simulink model "Heli_LQR2"  (Simulink 6.3)
settings: Solver=ode1  SolverMode=SingleTasking  StartTime=0.0  StopTime=inf  FixedStep=0.001  RelTol=1e-3
values from neighbouring files (symbols this model uses):
  g = 9.81    [setup_heli_LQR_instructor.m]    (also in setup_heli_LQR_parameters.m)
  h = 0.0139    [setup_heli_LQR_instructor.m]    (also in setup_heli_LQR_parameters.m)
  INT_JOYSTICK_SAT_LOWER = theta_0 * 180 / pi    (= -30)    [setup_heli_LQR_instructor.m]    (also in setup_heli_LQR_parameters.m)
  INT_JOYSTICK_SAT_UPPER = abs(theta_0)  * 180 / pi    [setup_heli_LQR_instructor.m]    (also in setup_heli_LQR_parameters.m)
  JOYSTICK_X_DZ = 0.25    [setup_heli_LQR_instructor.m]    (also in setup_heli_LQR_parameters.m)
  JOYSTICK_Y_DZ = 0.25    [setup_heli_LQR_instructor.m]    (also in setup_heli_LQR_parameters.m)
  K_CABLE_P = 5    [setup_heli_LQR_instructor.m]    (also in setup_heli_LQR_parameters.m)
  K_CABLE_Y = 3    [setup_heli_LQR_instructor.m]    (also in setup_heli_LQR_parameters.m)
  K_EC_P = - 2 * pi / ( 4 * 1024 )    (= -0.00153398078789)    [setup_heli_LQR_instructor.m]    (also in setup_heli_LQR_parameters.m)
  K_EC_Y = 2 * pi / ( 8 * 1024 )    (= 0.000766990393943)    [setup_heli_LQR_instructor.m]    (also in setup_heli_LQR_parameters.m)
  K_JOYSTICK_X = 85    [setup_heli_LQR_instructor.m]    (also in setup_heli_LQR_parameters.m)
  K_JOYSTICK_Y = 85    [setup_heli_LQR_instructor.m]    (also in setup_heli_LQR_parameters.m)
  K_pp = 0.185*0.20962    (= 0.0387797)    [setup_heli_LQR_instructor.m]    (also in setup_heli_LQR_parameters.m)
  K_py = 0.0041362    [setup_heli_LQR_instructor.m]    (also in setup_heli_LQR_parameters.m)
  K_yp = 0.0083316    [setup_heli_LQR_instructor.m]    (also in setup_heli_LQR_parameters.m)
  K_yy = 0.185*0.050271    (= 0.009300135)    [setup_heli_LQR_instructor.m]    (also in setup_heli_LQR_parameters.m)
  Ki = lqr(a,b,Qi,R)    [setup_heli_LQR_instructor.m]
  m_heli = 1.326    [setup_heli_LQR_instructor.m]    (also in setup_heli_LQR_parameters.m)
  Rc = 0.0094    [setup_heli_LQR_instructor.m]    (also in setup_heli_LQR_parameters.m)
  SAT_INT_ERR_PITCH = 20    [setup_heli_LQR_instructor.m]    (also in setup_heli_LQR_parameters.m)
  SAT_INT_ERR_YAW = 20    [setup_heli_LQR_instructor.m]    (also in setup_heli_LQR_parameters.m)
  theta_0 = -30*pi/180    (= -0.523598775598)    [setup_heli_LQR_instructor.m]    (also in setup_heli_LQR_parameters.m)
  Tr_p = 1    [setup_heli_LQR_instructor.m]    (also in setup_heli_LQR_parameters.m)
  Tr_y = 1    [setup_heli_LQR_instructor.m]    (also in setup_heli_LQR_parameters.m)
  VMAX_DAC = 10    [setup_heli_LQR_instructor.m]    (also in setup_heli_LQR_parameters.m)
  VMAX_UPM_P = 24    [setup_heli_LQR_instructor.m]    (also in setup_heli_LQR_parameters.m)
  VMAX_UPM_Y = 15    [setup_heli_LQR_instructor.m]    (also in setup_heli_LQR_parameters.m)
  wcf = 2 * pi * 20    (= 125.663706144)    [setup_heli_LQR_instructor.m]    (also in setup_heli_LQR_parameters.m)
  zetaf = 0.85    [setup_heli_LQR_instructor.m]    (also in setup_heli_LQR_parameters.m)
undefined symbols (not defined in the file or in its folder): Joystick, q_modules3
libraries: qctools x3
settings Model: LastModifiedBy=localadmin  ExtModeArmWhenConnect=off  BufferReuse=off  StrictBusMsg=None
settings ConfigSet: SimulationMode=external
settings OptimizationCC: BooleanDataType=off  InlineInvariantSignals=on  OptimizeBlockIOStorage=off  BufferReuse=off  ExpressionFolding=off  LocalBlockOutputs=off
settings RTWCC: SystemTargetFile=wincon.tlc  MakeCommand=make_wc  TemplateMakefile=wc_default_tmf  Description=WinCon Target  ProcessScript=wincon_make_rtw_hook
settings STFCustomTargetCC: TargetFcnLib=ansi_tfl_tmw.mat  GenFloatMathFcnCalls=ANSI_C  ModelReferenceCompliant=off  SystemTargetFile=wincon.tlc
settings GRTTargetCC: ModelReferenceCompliant=off  MatFileLogging=off  ExtMode=on  ExtModeTransport=2  ExtModeMexFile=wc_comm
settings CustomProperty: Value=on

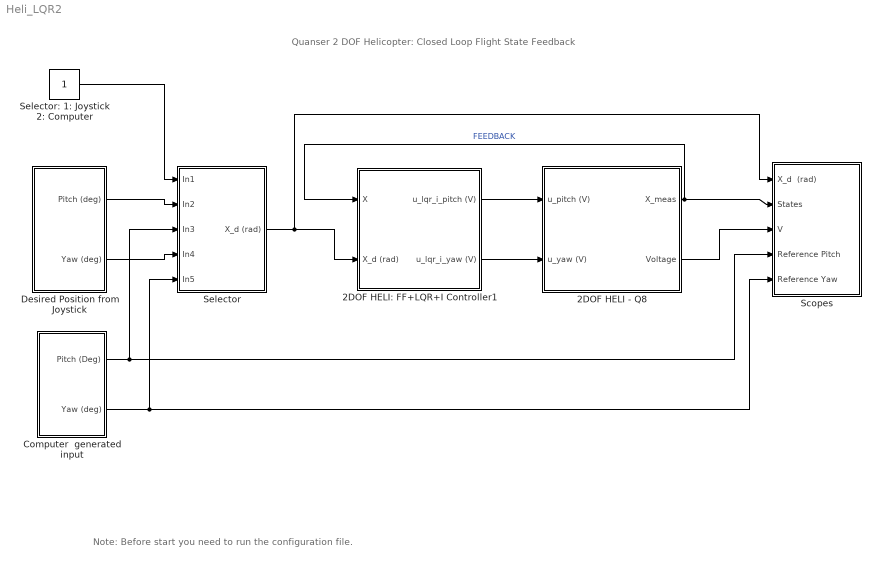
== system Heli_LQR2 ==
  note: Quanser 2 DOF Helicopter:
      | Closed Loop Flight
      | State Feedback
  note: Note: Before start you need to run the configuration file.
  2DOF HELI - Q8 : Subsystem  AncestorBlock=heli_2d_lib/2DOF HELI - Q8
  2DOF HELI: FF+LQR+I Controller1 : Subsystem  AncestorBlock=heli_2d_lib/2DOF HELI: FF+LQR+I Controller
  Computer  generated input : Subsystem
  Desired Position from Joystick : Subsystem  AncestorBlock=q_modules3/Joystick
  Scopes : Subsystem
  Selector : Subsystem
  Selector: 1: Joystick 2: Computer : Constant
  wires:
  2DOF HELI - Q8/1(X_meas) -> Scopes/2(States), 2DOF HELI: FF+LQR+I Controller1/1(X)  "FEEDBACK"
  2DOF HELI: FF+LQR+I Controller1/1(u_lqr_i_pitch (V)) -> 2DOF HELI - Q8/1(u_pitch (V))
  2DOF HELI: FF+LQR+I Controller1/2(u_lqr_i_yaw (V)) -> 2DOF HELI - Q8/2(u_yaw (V))
  Desired Position from Joystick/1(Pitch (deg)) -> Selector/2(In2)
  Computer  generated input/1(Pitch (Deg)) -> Selector/3(In3), Scopes/4(Reference Pitch)
  Desired Position from Joystick/2(Yaw (deg)) -> Selector/4(In4)
  Computer  generated input/2(Yaw (deg)) -> Selector/5(In5), Scopes/5(Reference Yaw)
  Selector: 1: Joystick 2: Computer/1 -> Selector/1(In1)
  Selector/1(X_d (rad)) -> Scopes/1(X_d  (rad)), 2DOF HELI: FF+LQR+I Controller1/2(X_d (rad))
  2DOF HELI - Q8/2(Voltage) -> Scopes/3(V)

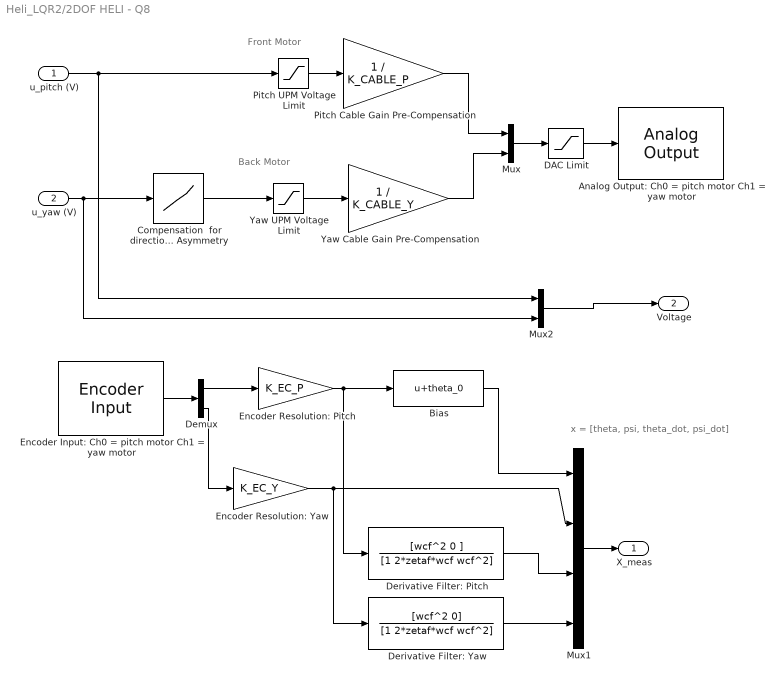
== system Heli_LQR2/2DOF HELI - Q8 ==
  note: Back Motor
  note: Front Motor
  note: x = [theta, psi, theta_dot, psi_dot]
  u_pitch (V) : Inport
  u_yaw (V) : Inport  Port=2
  Analog Output: Ch0 = pitch motor Ch1 = yaw motor : qctools/Quanser Consulting Q8 Series/Analog Output  boardNumber=0  channels=[0,1]  modesVect=0  rangesVect=10  initialVect=0  finalVect=0  sampleTime=-1  inputVolts=on  simulationOutput=off
  Bias : Bias  Bias=theta_0
  "Compensation  for direction Asymmetry " : Lookup  InputValues="[-[12.5  10 7.5]  0  [7.5 10  12.5 15] ]"  OutputValues="[-[12.5  10 7.5] *.4 0  [7.5 10  12.5 15] ]"
  DAC Limit : Saturate  UpperLimit=VMAX_DAC  LowerLimit=- VMAX_DAC
  Demux : Demux  Outputs=2
  Derivative Filter: Pitch : TransferFcn  Numerator=[wcf^2 0 ]  Denominator=[1 2*zetaf*wcf wcf^2]
  Derivative Filter: Yaw : TransferFcn  Numerator=[wcf^2 0]  Denominator=[1 2*zetaf*wcf wcf^2]
  Encoder Input: Ch0 = pitch motor Ch1 = yaw motor : qctools/Quanser Consulting Q8 Series/Encoder Input  boardNumber=0  channels=[0,1]  initial=0  preserveCounts=off  sampleTime=default_sample_time  quadratureStr=4X  modeStr=Normal  flagString=FLG1 is IDX and FLG2 is E  prescale=1  frequency=16666666.6667  bcd=off  enableIndex=on  synchronousIndex=on  indexPolarity=on  reloadOnIndex=off  simulationInput=off
  "Encoder Resolution: Pitch " : Gain  Gain=K_EC_P
  Encoder Resolution: Yaw : Gain  Gain=K_EC_Y
  Mux : Mux  Inputs=2
  Mux1 : Mux
  Mux2 : Mux  Inputs=2
  Pitch Cable Gain Pre-Compensation : Gain  Gain=1 / K_CABLE_P  SaturateOnIntegerOverflow=on
  Pitch UPM Voltage Limit : Saturate  UpperLimit=VMAX_UPM_P  LowerLimit=- VMAX_UPM_P
  Yaw Cable Gain Pre-Compensation : Gain  Gain=1 / K_CABLE_Y  SaturateOnIntegerOverflow=on
  Yaw UPM Voltage Limit : Saturate  UpperLimit=VMAX_UPM_Y  LowerLimit=- VMAX_UPM_Y
  X_meas : Outport
  Voltage : Outport  Port=2
  wires:
  Encoder Resolution: Yaw/1 -> Mux1/2, Derivative Filter: Yaw/1
  Yaw Cable Gain Pre-Compensation/1 -> Mux/2
  Pitch Cable Gain Pre-Compensation/1 -> Mux/1
  Mux1/1 -> X_meas/1
  u_pitch (V)/1 -> Pitch UPM Voltage Limit/1, Mux2/1
  Yaw UPM Voltage Limit/1 -> Yaw Cable Gain Pre-Compensation/1
  Pitch UPM Voltage Limit/1 -> Pitch Cable Gain Pre-Compensation/1
  DAC Limit/1 -> Analog Output: Ch0 = pitch motor Ch1 = yaw motor/1
  Mux/1 -> DAC Limit/1
  Demux/1 -> "Encoder Resolution: Pitch "/1
  "Encoder Resolution: Pitch "/1 -> Bias/1, Derivative Filter: Pitch/1
  Encoder Input: Ch0 = pitch motor Ch1 = yaw motor/1 -> Demux/1
  Demux/2 -> Encoder Resolution: Yaw/1
  Bias/1 -> Mux1/1
  Derivative Filter: Pitch/1 -> Mux1/3
  Derivative Filter: Yaw/1 -> Mux1/4
  "Compensation  for direction Asymmetry "/1 -> Yaw UPM Voltage Limit/1
  u_yaw (V)/1 -> "Compensation  for direction Asymmetry "/1, Mux2/2
  Mux2/1 -> Voltage/1

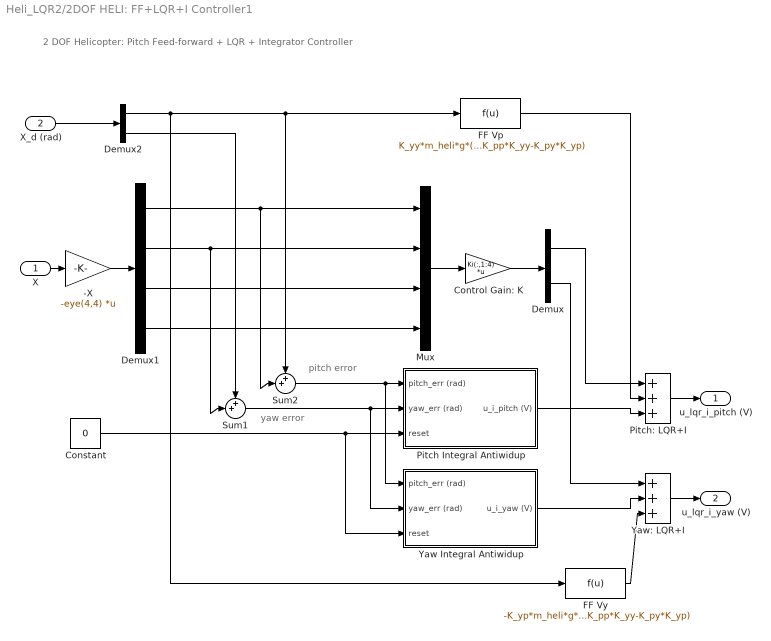
== system Heli_LQR2/2DOF HELI: FF+LQR+I Controller1 ==
  note: yaw error
  note: pitch error
  note: 2 DOF Helicopter:
      | Pitch Feed-forward + LQR + Integrator Controller
  X : Inport
  X_d (rad) : Inport  Port=2
  -X : Gain  Gain=-eye(4,4)  Multiplication=Matrix(K*u)
  Constant : Constant  Value=0
  Control Gain: K : Gain  Gain=Ki(:,1:4)  Multiplication=Matrix(K*u)
  Demux : Demux  Outputs=2
  Demux1 : Demux
  Demux2 : Demux  Outputs=2
  FF Vp : Fcn  Expr="K_yy*m_heli*g*(h*sin(u[1]) + Rc*cos(u[1]))  /  (K_pp*K_yy-K_py*K_yp)"
  FF Vy : Fcn  Expr="-K_yp*m_heli*g*(h*sin(u[1]) + Rc*cos(u[1]))  /  (K_pp*K_yy-K_py*K_yp)"
  Mux : Mux
  Pitch Integral Antiwidup : Subsystem  AncestorBlock=heli_2d_lib/2DOF HELI: FF+LQR+I Controller/Yaw Integral Antiwidup
  Pitch: LQR+I : Sum  Inputs=+++  OutScaling=2^-10
  Sum1 : Sum  Inputs=++|
  Sum2 : Sum  Inputs=++|
  Yaw Integral Antiwidup : Subsystem
  Yaw: LQR+I : Sum  Inputs=+++  OutScaling=2^-10
  u_lqr_i_pitch (V) : Outport
  u_lqr_i_yaw (V) : Outport  Port=2
  wires:
  Constant/1 -> Pitch Integral Antiwidup/3(reset), Yaw Integral Antiwidup/3(reset)
  Demux1/2 -> Sum1/2, Mux/2
  Demux2/2 -> Sum1/1
  Demux2/1 -> Sum2/1, FF Vp/1, FF Vy/1
  X_d (rad)/1 -> Demux2/1
  Yaw Integral Antiwidup/1(u_i_yaw (V)) -> Yaw: LQR+I/2
  Demux/2 -> Yaw: LQR+I/1
  Yaw: LQR+I/1 -> u_lqr_i_yaw (V)/1
  Pitch: LQR+I/1 -> u_lqr_i_pitch (V)/1
  Demux/1 -> Pitch: LQR+I/2
  Pitch Integral Antiwidup/1(u_i_pitch (V)) -> Pitch: LQR+I/3
  FF Vp/1 -> Pitch: LQR+I/1
  Sum2/1 -> Pitch Integral Antiwidup/1(pitch_err (rad)), Yaw Integral Antiwidup/1(pitch_err (rad))
  Demux1/1 -> Sum2/2, Mux/1
  X/1 -> -X/1
  Sum1/1 -> Pitch Integral Antiwidup/2(yaw_err (rad)), Yaw Integral Antiwidup/2(yaw_err (rad))
  -X/1 -> Demux1/1
  Control Gain: K/1 -> Demux/1
  Mux/1 -> Control Gain: K/1
  Demux1/3 -> Mux/3
  Demux1/4 -> Mux/4
  FF Vy/1 -> Yaw: LQR+I/3

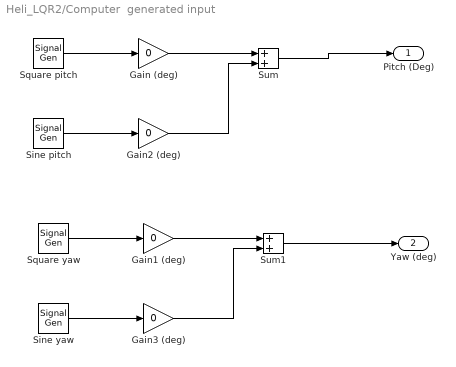
== system Heli_LQR2/Computer  generated input ==
  Gain (deg) : Gain  Gain=0
  Gain1 (deg) : Gain  Gain=0
  Gain2 (deg) : Gain  Gain=0
  Gain3 (deg) : Gain  Gain=0
  Sine pitch : SignalGenerator  Frequency=1/30
  Sine yaw : SignalGenerator  Frequency=.02
  Square pitch : SignalGenerator  WaveForm=square  Frequency=1/30
  Square yaw : SignalGenerator  WaveForm=square  Frequency=1/60*2
  Sum : Sum
  Sum1 : Sum
  Pitch (Deg) : Outport
  Yaw (deg) : Outport  Port=2
  wires:
  Square pitch/1 -> Gain (deg)/1
  Gain (deg)/1 -> Sum/1
  Sum/1 -> Pitch (Deg)/1
  Sine pitch/1 -> Gain2 (deg)/1
  Gain2 (deg)/1 -> Sum/2
  Square yaw/1 -> Gain1 (deg)/1
  Gain1 (deg)/1 -> Sum1/1
  Sum1/1 -> Yaw (deg)/1
  Sine yaw/1 -> Gain3 (deg)/1
  Gain3 (deg)/1 -> Sum1/2

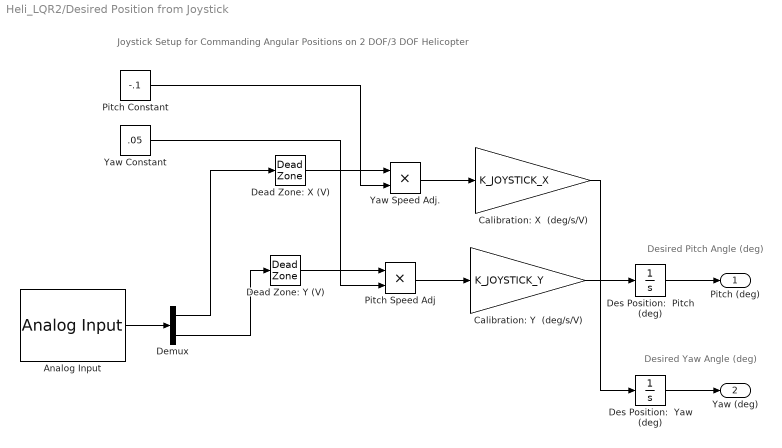
== system Heli_LQR2/Desired Position from Joystick ==
  note: Joystick Setup for Commanding Angular Positions on 2 DOF/3 DOF Helicopter
  note: Desired Yaw Angle (deg)
  note: Desired Pitch Angle (deg)
  Analog Input : qctools/Quanser Consulting Q8 Series/Analog Input  boardNumber=0  channels=[2 3]  sampleTime=default_sample_time  useBusy=on  simultaneous=on  outputVolts=on  simulationInput=off
  Calibration: X  (deg/s/V) : Gain  Gain=K_JOYSTICK_X
  Calibration: Y  (deg/s/V) : Gain  Gain=K_JOYSTICK_Y
  Dead Zone: X (V) : DeadZone  LowerValue=-JOYSTICK_X_DZ  UpperValue=JOYSTICK_X_DZ  SaturateOnIntegerOverflow=on
  Dead Zone: Y (V) : DeadZone  LowerValue=-JOYSTICK_Y_DZ  UpperValue=JOYSTICK_Y_DZ  SaturateOnIntegerOverflow=on
  Demux : Demux  Outputs=2
  Des Position:  Pitch (deg) : Integrator  InitialCondition=theta_0*180/pi  LimitOutput=on  UpperSaturationLimit=INT_JOYSTICK_SAT_UPPER  LowerSaturationLimit=INT_JOYSTICK_SAT_LOWER
  Des Position:  Yaw (deg) : Integrator  UpperSaturationLimit=180  LowerSaturationLimit=-180
  Pitch Constant : Constant  Value=-.1
  Pitch Speed Adj : Product  RndMeth=Zero
  Yaw Constant : Constant  Value=.05
  Yaw Speed Adj. : Product  RndMeth=Zero
  Pitch (deg) : Outport
  Yaw (deg) : Outport  Port=2
  wires:
  Yaw Constant/1 -> Pitch Speed Adj/2
  Demux/2 -> Dead Zone: Y (V)/1
  Demux/1 -> Dead Zone: X (V)/1
  Pitch Constant/1 -> Yaw Speed Adj./2
  Analog Input/1 -> Demux/1
  Calibration: Y  (deg/s/V)/1 -> Des Position:  Pitch (deg)/1
  Pitch Speed Adj/1 -> Calibration: Y  (deg/s/V)/1
  Yaw Speed Adj./1 -> Calibration: X  (deg/s/V)/1
  Dead Zone: Y (V)/1 -> Pitch Speed Adj/1
  Dead Zone: X (V)/1 -> Yaw Speed Adj./1
  Calibration: X  (deg/s/V)/1 -> Des Position:  Yaw (deg)/1
  Des Position:  Yaw (deg)/1 -> Yaw (deg)/1
  Des Position:  Pitch (deg)/1 -> Pitch (deg)/1

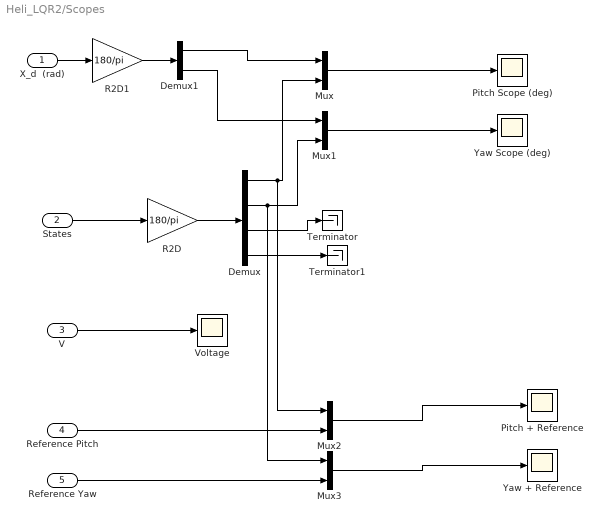
== system Heli_LQR2/Scopes ==
  X_d  (rad) : Inport
  States : Inport  Port=2
  V : Inport  Port=3
  Reference Pitch : Inport  Port=4
  Reference Yaw : Inport  Port=5
  Demux : Demux
  Demux1 : Demux  Outputs=2
  Mux{,1..3} (4 alike) : Mux  Inputs=2
  Pitch + Reference : Scope
  Pitch Scope (deg) : Scope
      settings: SaveName=ScopeData6
  R2D : Gain  Gain=180/pi
  R2D1 : Gain  Gain=180/pi
  Terminator : Terminator
  Terminator1 : Terminator
  Voltage : Scope
  Yaw + Reference : Scope
      settings: SaveName=ScopeData2
  Yaw Scope (deg) : Scope
      settings: SaveName=ScopeData7
  wires:
  Demux/1 -> Mux/2, Mux2/1
  States/1 -> R2D/1
  R2D/1 -> Demux/1
  Mux/1 -> Pitch Scope (deg)/1
  Mux1/1 -> Yaw Scope (deg)/1
  Demux/2 -> Mux1/2, Mux3/1
  Demux/3 -> Terminator/1
  Demux/4 -> Terminator1/1
  X_d  (rad)/1 -> R2D1/1
  Demux1/1 -> Mux/1
  Demux1/2 -> Mux1/1
  R2D1/1 -> Demux1/1
  V/1 -> Voltage/1
  Reference Pitch/1 -> Mux2/2
  Reference Yaw/1 -> Mux3/2
  Mux2/1 -> Pitch + Reference/1
  Mux3/1 -> Yaw + Reference/1

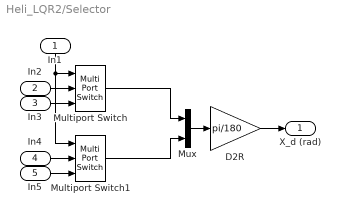
== system Heli_LQR2/Selector ==
  In1 : Inport  Orientation=down
  In2 : Inport  Port=2
  In3 : Inport  Port=3
  In4 : Inport  Port=4
  In5 : Inport  Port=5
  D2R : Gain  Gain=pi/180
  Multiport Switch : MultiPortSwitch  Inputs=2
  Multiport Switch1 : MultiPortSwitch  Inputs=2
  Mux : Mux  Inputs=2
  X_d (rad) : Outport
  wires:
  In1/1 -> Multiport Switch/1, Multiport Switch1/1
  In2/1 -> Multiport Switch/2
  Multiport Switch/1 -> Mux/1
  In3/1 -> Multiport Switch/3
  In4/1 -> Multiport Switch1/2
  Multiport Switch1/1 -> Mux/2
  In5/1 -> Multiport Switch1/3
  Mux/1 -> D2R/1
  D2R/1 -> X_d (rad)/1

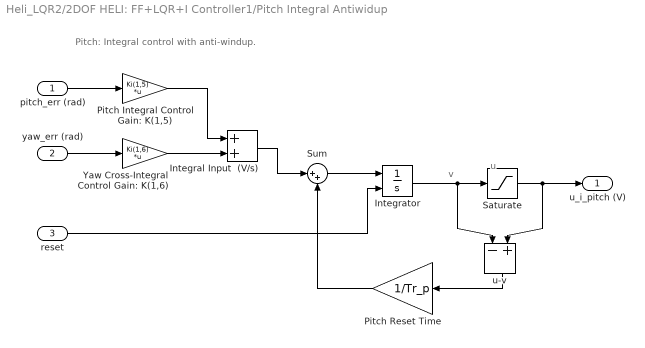
== system Heli_LQR2/2DOF HELI: FF+LQR+I Controller1/Pitch Integral Antiwidup ==
  note: Pitch: Integral control with anti-windup.
  note: v
  note: u
  pitch_err (rad) : Inport
  yaw_err (rad) : Inport  Port=2
  reset : Inport  Port=3
  Integral Input  (V/s) : Sum  OutScaling=2^-10
  Integrator : Integrator  ExternalReset=rising
  Pitch Integral Control Gain: K(1,5) : Gain  Gain=Ki(1,5)  Multiplication=Matrix(K*u)
  Pitch Reset Time : Gain  Orientation=left  Gain=1/Tr_p
  Saturate : Saturate  UpperLimit=SAT_INT_ERR_PITCH  LowerLimit=-SAT_INT_ERR_PITCH
  Sum : Sum  Inputs=|++
  Yaw Cross-Integral Control Gain: K(1,6) : Gain  Gain=Ki(1,6)  Multiplication=Matrix(K*u)
  u-v : Sum  Orientation=down  Inputs=-+  OutScaling=2^-10
  u_i_pitch (V) : Outport
  wires:
  Integral Input  (V/s)/1 -> Sum/1
  Yaw Cross-Integral Control Gain: K(1,6)/1 -> Integral Input  (V/s)/2
  Pitch Integral Control Gain: K(1,5)/1 -> Integral Input  (V/s)/1
  yaw_err (rad)/1 -> Yaw Cross-Integral Control Gain: K(1,6)/1
  reset/1 -> Integrator/2
  Pitch Reset Time/1 -> Sum/2
  Sum/1 -> Integrator/1
  u-v/1 -> Pitch Reset Time/1
  Saturate/1 -> u-v/2, u_i_pitch (V)/1
  Integrator/1 -> Saturate/1, u-v/1
  pitch_err (rad)/1 -> Pitch Integral Control Gain: K(1,5)/1

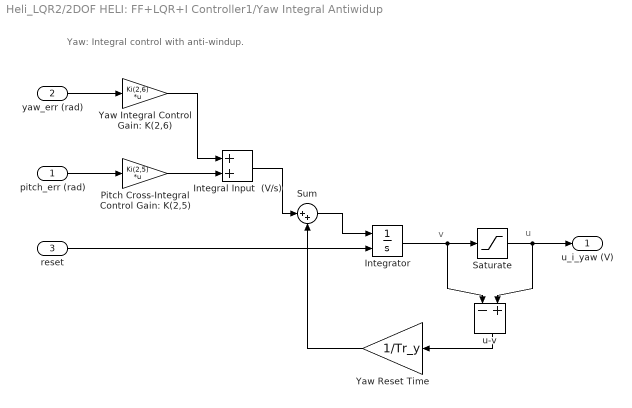
== system Heli_LQR2/2DOF HELI: FF+LQR+I Controller1/Yaw Integral Antiwidup ==
  note: Yaw: Integral control with anti-windup.
  note: u
  note: v
  pitch_err (rad) : Inport
  yaw_err (rad) : Inport  Port=2
  reset : Inport  Port=3
  Integral Input  (V/s) : Sum  OutScaling=2^-10
  Integrator : Integrator  ExternalReset=rising
  Pitch Cross-Integral Control Gain: K(2,5) : Gain  Gain=Ki(2,5)  Multiplication=Matrix(K*u)
  Saturate : Saturate  UpperLimit=SAT_INT_ERR_YAW  LowerLimit=-SAT_INT_ERR_YAW
  Sum : Sum  Inputs=|++
  Yaw Integral Control Gain: K(2,6) : Gain  Gain=Ki(2,6)  Multiplication=Matrix(K*u)
  Yaw Reset Time : Gain  Orientation=left  Gain=1/Tr_y
  u-v : Sum  Orientation=down  Inputs=-+  OutScaling=2^-10
  u_i_yaw (V) : Outport
  wires:
  Integral Input  (V/s)/1 -> Sum/1
  Pitch Cross-Integral Control Gain: K(2,5)/1 -> Integral Input  (V/s)/2
  Yaw Integral Control Gain: K(2,6)/1 -> Integral Input  (V/s)/1
  pitch_err (rad)/1 -> Pitch Cross-Integral Control Gain: K(2,5)/1
  reset/1 -> Integrator/2
  yaw_err (rad)/1 -> Yaw Integral Control Gain: K(2,6)/1
  Integrator/1 -> u-v/1, Saturate/1
  Saturate/1 -> u_i_yaw (V)/1, u-v/2
  u-v/1 -> Yaw Reset Time/1
  Sum/1 -> Integrator/1
  Yaw Reset Time/1 -> Sum/2
